simulink library "Data_from_File"  (R2018b)
settings: Solver=ode45  StartTime=0.0  StopTime=10.0  RelTol=1e-3  EnableMultiTasking=on
undefined symbols (not defined in the file): path_carnot
settings Model: Creator=lena.frank  LastModifiedBy=P41573
settings DataIOCC: LimitDataPoints=on  SaveFormat=Array  SignalLoggingSaveFormat=ModelDataLogs
settings OptimizationCC: ExpressionDepthLimit=2147483647  LifeSpan=inf
settings DebuggingCC: UnderspecifiedInitializationDetection=Classic  MergeDetectMultiDrivingBlocksExec=none  SolverPrmCheckMsg=warning  FcnCallInpInsideContextMsg=warning  StateNameClashWarn=warning  SFUnexpectedBacktrackingDiag=warning  SFNoUnconditionalDefaultTransitionDiag=warning  SFExecutionAtInitializationDiag=none
settings HardwareCC: ProdBitPerPointer=32  ProdBitPerSizeT=32  ProdBitPerPtrDiffT=32  ProdLargestAtomicFloat=None  ProdIntDivRoundTo=Undefined  ProdEndianess=Unspecified  ProdWordSize=32  ProdHWDeviceType=32-bit Generic
settings ModelReferenceCC: PropagateSignalLabelsOutOfModel=off
settings SFSimCC: SimUseLocalCustomCode=off
settings RTWCC: RTWUseLocalCustomCode=off
settings CodeAppCC: StateflowObjectComments=on
settings GRTTargetCC: TargetLangStandard=C89/C90 (ANSI)  GeneratePreprocessorConditionals=Disable all  CombineOutputUpdateFcns=off  GRTInterface=on
settings ConfigComp: CovMetricSettings=dw  CovHtmlReporting=on  CovSaveCumulativeToWorkspaceVar=on  CovSaveSingleToWorkspaceVar=on  CovExternalEMLEnable=off

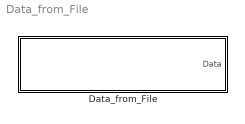
== system Data_from_File ==
  Data_from_File : Subsystem  mask(Data from File){PathName=path_carnot('data'), FileName='ElectricProfile_SHC_IEA_Task44.mat', UserParam=off, DataName=DataName, t_sample=60}
      mask prompts: PathName "Path"; FileName "File"; UserParam "Edit file and path"; DataName "Variable name"; t_sample "Timestep in data"
      mask help:
      | Loads data in a variable in the workspace. A "From Workspace" block in the subsystem uses this variable. The data matrix must contain the time (in s) as a first column. A Unit-Delay with the "Timestep in data" forces the model to a maximum timestep equal to the data timestep.
      | Buttons in the "Picking a file" opens a window to chose a data file:
      | 1) "From selected path"  from the path shown  in the "Selection" frame.
      | 2) "Carnot public data" from the public data folder in Carnot.
      | 3) "Carnot internal data" from the internal data folder in Carnot.
      | You edit "File" and "Path" after activating the checkbox. Enter 'current' as path and the choice will start in the current Matlab directory.
      | You can use the createDatafile.m function to create the files from .csv or other inputs.
      mask init:
      | [ok,DataName,t_sample] = CarnotCallbacks_Data_from_File('LoadData', ...
      |     gcbh, PathName, FileName);
      mask Help: web(fullfile(path_carnot('help'),'Data_from_file.html'),'-helpbrowser')
      mask Callback UserParam: ok = CarnotCallbacks_Data_from_File('UserMaskEnable',gcbh);
      mask DialogControl ParameterGroupVar Prompt: Picking a file
      mask DialogControl Control2 Prompt: From selected path
      mask DialogControl Control2 Callback: ok = CarnotCallbacks_Data_from_File('GetFilename',gcbh, 'selected');
      mask DialogControl Control3 Prompt: Carnot public data
      mask DialogControl Control3 Callback: ok = CarnotCallbacks_Data_from_File('GetFilename',gcbh, 'public');
      mask DialogControl Control4 Prompt: Carnot internal data
      mask DialogControl Control4 Callback: ok = CarnotCallbacks_Data_from_File('GetFilename',gcbh, 'internal');
      mask DialogControl Container3 Prompt: Selection
      mask Display: disp(['Data file:\n', FileName(1:end-4)])

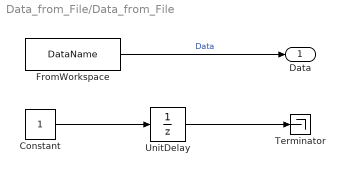
== system Data_from_File/Data_from_File ==
  Constant : Constant
  FromWorkspace : FromWorkspace  VariableName=DataName  SampleTime=0  OutputAfterFinalValue=Holding final value
  Terminator : Terminator
  UnitDelay : UnitDelay  SampleTime=t_sample
  Data : Outport
  wires:
  UnitDelay/1 -> Terminator/1
  Constant/1 -> UnitDelay/1
  FromWorkspace/1 -> Data/1  "Data"
